simulink model "deflectionTestSim"  (R2022a)
settings: Solver=FixedStepAuto  StartTime=0.0  StopTime=50  RelTol=1e-3
libraries: aru_toolbox x2
settings Model: Creator=Mechatronics  LastModifiedBy=Mechatronics
settings SolverCC: ConcurrentTasks=on  PositivePriorityOrder=on
settings OptimizationCC: BlockReduction=off  OptimizeBlockIOStorage=off
settings DebuggingCC: TasksWithSamePriorityMsg=none
settings HardwareCC: ProdBitPerLong=64  ProdLongLongMode=on  ProdHWDeviceType=Intel->x86-64 (Linux 64)
settings RTWCC: Description=Simulink Real-Time  SystemTargetFile=slrealtime.tlc  TemplateMakefile=slrealtime_default_tmf  Toolchain=Simulink Real-Time Toolchain  BuildConfiguration=Faster Runs  CodeExecutionProfiling=on  TargetLang=C++

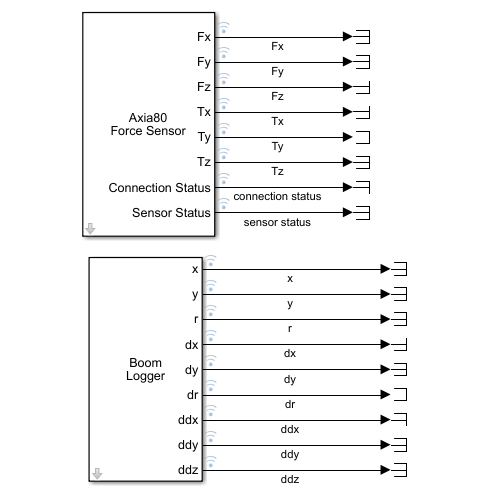
[thumbnail: Simulink's stored preview of the top-level diagram]
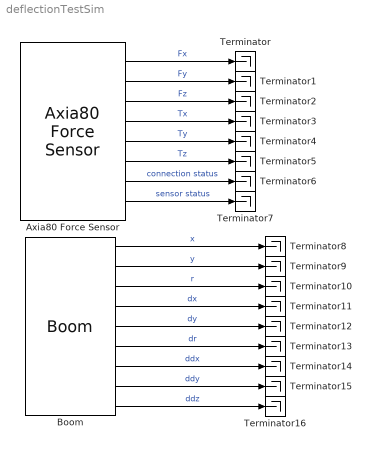
== system deflectionTestSim ==
  Axia80 Force Sensor : aru_toolbox/Axia80 Force Sensor  resetBias=on  calibrationRangeParam=Range 0 (500N Fxy, 900N Fz, 20Nm Txyz)  sampleRateParam=975Hz  filterParam=No filtering (200Hz @ 0.5kHz, 350Hz @ 1kHz, 500Hz @ 2kHz, 1000Hz @ 4kHz)
      settings: SourceProductName=ARU Toolbox
  Boom : aru_toolbox/Boom  ts=0.001
      link override Serial Read HW FIFO: pciSlot=-1
      link override Serial Setup: pciSlot=-1
      settings: SourceProductName=ARU Toolbox
  Terminator{,1..16} (17 alike) : Terminator
  wires:
  Axia80 Force Sensor/1 -> Terminator/1  "Fx"
  Axia80 Force Sensor/2 -> Terminator1/1  "Fy"
  Axia80 Force Sensor/3 -> Terminator2/1  "Fz"
  Axia80 Force Sensor/4 -> Terminator3/1  "Tx"
  Axia80 Force Sensor/5 -> Terminator4/1  "Ty"
  Axia80 Force Sensor/6 -> Terminator5/1  "Tz"
  Axia80 Force Sensor/7 -> Terminator6/1  "connection status"
  Axia80 Force Sensor/8 -> Terminator7/1  "sensor status"
  Boom/8 -> Terminator15/1  "ddy"
  Boom/1 -> Terminator8/1  "x"
  Boom/2 -> Terminator9/1  "y"
  Boom/3 -> Terminator10/1  "r"
  Boom/4 -> Terminator11/1  "dx"
  Boom/5 -> Terminator12/1  "dy"
  Boom/6 -> Terminator13/1  "dr"
  Boom/7 -> Terminator14/1  "ddx"
  Boom/9 -> Terminator16/1  "ddz"
